simulink model "NEW_QUAD_realtime_DC_motor_test"  (R2021a)
settings: Solver=VariableStepAuto  StartTime=0.0  StopTime=10.0  RelTol=1e-3
values from neighbouring files (symbols this model uses):
  Ts = 0.1    [ddpg_setup_file.m]    (also in realtime_testing_ddpg_3000_agent_100rpm(31stMay)_WS.mat = 0.01)
undefined symbols (not defined in the file or in its folder): DiscIntNeverNeededParam
libraries: simulink x2, rllib x1, aerolibanimutils x1
settings Model: Creator=SHRENI MALYALA  LastModifiedBy=SHRENI MALYALA

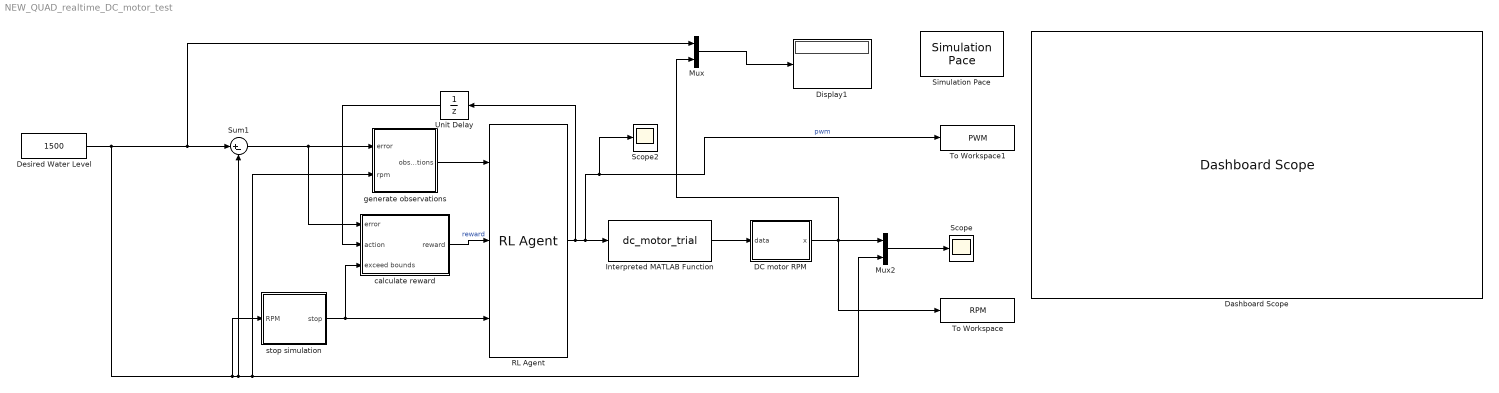
== system NEW_QUAD_realtime_DC_motor_test ==
  "DC motor RPM " : MATLAB Function  TreatAsAtomicUnit=on
  Dashboard Scope : DashboardScope  Ymin=0  Ymax=4000
  Desired Water Level : Constant  Value=1500
  Display1 : Display
  Interpreted MATLAB Function : MATLABFcn  MATLABFcn=dc_motor_trial  OutputDimensions=[1,2]  Output1D=off
  Mux : Mux  Inputs=2
  Mux2 : Mux  Inputs=2
  RL Agent : rllib/RL Agent  Agent=agent  ExternalActionAsInput=off  ProvideCumRwd=off  TreatAsDirectFeedthrough=on
  Scope : Scope
  Scope2 : Scope
  Simulation Pace : aerolibanimutils/Simulation Pace  SimulationPace=1  SleepMode=MATLAB Thread  OutputPaceError=off  SampleTime=0.01
  Sum1 : Sum  Inputs=|+-  SaturateOnIntegerOverflow=on
  To Workspace : ToWorkspace  VariableName=RPM  SampleTime=0.01
  To Workspace1 : ToWorkspace  VariableName=PWM  SaveFormat=Timeseries  SampleTime=0.01
  Unit Delay : UnitDelay  SampleTime=-1  HasFrameUpgradeWarning=on
  calculate reward : Subsystem
  generate observations : Subsystem
  stop simulation : Subsystem
  wires:
  Unit Delay/1 -> calculate reward/2(action)
  RL Agent/1 -> Unit Delay/1, Interpreted MATLAB Function/1, Scope2/1, To Workspace1/1  "pwm"
  Mux/1 -> Display1/1
  stop simulation/1(stop) -> RL Agent/3, calculate reward/3(exceed bounds)
  calculate reward/1(reward) -> RL Agent/2  "reward"
  Sum1/1 -> calculate reward/1(error), generate observations/1(error)
  generate observations/1(observations) -> RL Agent/1
  Mux2/1 -> Scope/1
  Interpreted MATLAB Function/1 -> "DC motor RPM "/1(data)
  "DC motor RPM "/1(x) -> Mux/2, To Workspace/1, Mux2/1
  Desired Water Level/1 -> Sum1/2, generate observations/2(rpm), Mux2/2, stop simulation/1(RPM), Sum1/1, Mux/1

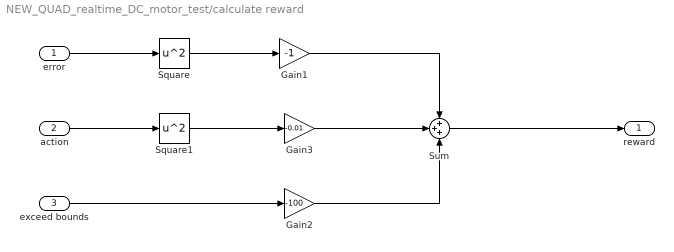
== system NEW_QUAD_realtime_DC_motor_test/calculate reward ==
  error : Inport
  action : Inport  Port=2
  exceed bounds : Inport  Port=3
  Gain1 : Gain  Gain=-1
  Gain2 : Gain  Gain=-100
  Gain3 : Gain  Gain=-0.01
  Square : Math  Operator=square  SaturateOnIntegerOverflow=on
  Square1 : Math  Operator=square  SaturateOnIntegerOverflow=on
  Sum : Sum  Inputs=+++  OutDataTypeStr=double
  reward : Outport  VectorParamsAs1DForOutWhenUnconnected=off
  wires:
  Sum/1 -> reward/1
  exceed bounds/1 -> Gain2/1
  action/1 -> Square1/1
  error/1 -> Square/1
  Square1/1 -> Gain3/1
  Square/1 -> Gain1/1
  Gain1/1 -> Sum/1
  Gain3/1 -> Sum/2
  Gain2/1 -> Sum/3

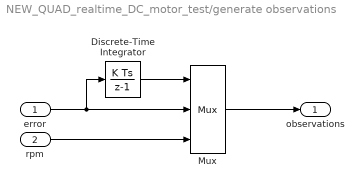
== system NEW_QUAD_realtime_DC_motor_test/generate observations ==
  error : Inport
  rpm : Inport  Port=2
  Discrete-Time Integrator : DiscreteIntegrator  SampleTime=Ts  ICPrevOutput=DiscIntNeverNeededParam  ICPrevScaledInput=DiscIntNeverNeededParam
  Mux : Mux  Inputs=3
  observations : Outport  VectorParamsAs1DForOutWhenUnconnected=off
  wires:
  rpm/1 -> Mux/3
  Discrete-Time Integrator/1 -> Mux/1
  error/1 -> Discrete-Time Integrator/1, Mux/2
  Mux/1 -> observations/1

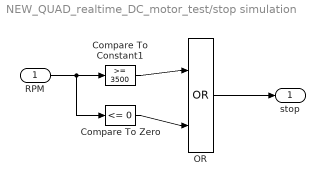
== system NEW_QUAD_realtime_DC_motor_test/stop simulation ==
  RPM : Inport
  Compare To Constant1 : simulink/Logic and Bit Operations/Compare To Constant  relop=>=  const=3500  OutDataTypeStr=boolean
  Compare To Zero : simulink/Logic and Bit Operations/Compare To Zero  relop=<=  OutDataTypeStr=boolean
  OR : Logic  Operator=OR  IconShape=distinctive  AllPortsSameDT=off  OutDataTypeStr=boolean
  stop : Outport  VectorParamsAs1DForOutWhenUnconnected=off
  wires:
  RPM/1 -> Compare To Zero/1, Compare To Constant1/1
  Compare To Zero/1 -> OR/2
  Compare To Constant1/1 -> OR/1
  OR/1 -> stop/1

== matlab function NEW_QUAD_realtime_DC_motor_test/DC motor RPM  ==
  data: data input; x output
function x  = PWM(data)

F = data(:,1)*256;
r = data(:,2);
x = (F+r)*8.982025;

end
